simulink model "filter_music"  (R2021a)
settings: Solver=FixedStepDiscrete  StartTime=0.0  StopTime=inf  RelTol=1e-3
undefined symbols (not defined in the file or in its folder): fdesignblkfcn, gcbh
libraries: dspfdesign x2, dspsnks4 x1, dspvision x1
(part 2 of 2)

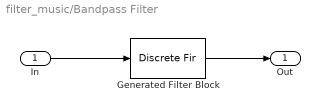
== system filter_music/Bandpass Filter ==
  In : Inport
  Generated Filter Block : DiscreteFir  Tag=BlockMethodSubSystem  Coefficients=[-0.000605180765563559896 -0.000235381781177703146 -0.000262859375971625413 -0.000278554889448817417 -0.000279923053767988173 -0.000265464035195501331 -0.000234716056378071693 -0.00018863467570875262 -0.000129411281477895067 -6.06366503102824512e-05 1.31467495266928401e-05 8.65511069714545132e-05 0.000154034385313488062 0.000210145628121449752 0.000250253378986492556 0.00027071164836725976 0.000269490837798465311 0.000246231290949470159 0.000202784352817899423 0.000143028939846710291 7.29851468422456316e-05 -4.77348731589156425e-08 -6.79070740966332198e-05 -0.000122541384684050962 -0.000155931925683581134 -0.000160955543706951999 -0.000132226172829594377 -6.83521227724636759e-05 2.96378115559616279e-05 0.000160133019832697597 0.000313569795262432708 0.000481870213809313969 0.000652141561601816229 0.000811036194270708792 0.000944251143223556614 0.00103811317126550613 0.00108045816269594945 0.00106184513278247605 0.000976405444503380244 0.00082256507615554122 0.000603383089157199072 0.000326581850271807439 4.30229332145489322e-06 -0.000347509148140041164 -0.000709960328759635549 -0.00106252114048841937 -0.00138437477114929076 -0.00165591825323341529 -0.00185992926996901738 -0.00198287607906476315 -0.00201592256171890302 -0.00195586315981783384 -0.00180507449704414048 -0.00157138964197742789 -0.00126771264216854322 -0.000911677520776701445 -0.000523426256061187674 -0.000124603742469066113 0.000262166881930523115 0.00061678380216169859 0.000920925730041676697 0.0011607996965117013 0.00132708911283209246 0.00141590960857993289 0.00142864204842689199 0.00137169545143854825 0.00125574284285703266 0.00109477510338883361 0.000904879511926304876 0.00070287872131849006 0.000504967982929463671 0.000325453791699786691 0.000175792867800047452 6.37979729521747317e-05 -6.78212542151071728e-06 -3.64090327009696142e-05 -2.93132352749527577e-05 7.10364132435301075e-06 6.31354581538463882e-05 0.000127627008729503587 0.000189328520858482891 0.000237969883486319108 0.000265138541684875443 0.000264854787163768164 0.000234581092845862979 0.00017485918044263192 8.92504407498085451e-05 -1.55906822884784904e-05 -0.000131442770007978067 -0.00024855850135476051 -0.000357255458734658665 -0.000448464748990436764 -0.000514815634287659135 -0.000551228314512786977 -0.000555453484683462984 -0.000528225669558642693 -0.000473150348547238578 -0.000396334954072101626 -0.000305796015337770548 -0.000210708853438425523 -0.00012045061728521669 -4.37072089313232244e-05 1.23630628756550677e-05 4.27142101961259989e-05 4.49781553983374631e-05 1.9660819291976721e-05 -2.99127335878764909e-05 -9.80525281223114018e-05 -0.000177090847882267245 -0.00025819999365800085 -0.000332283691101674156 -0.000390876997623911665 -0.000426702885764895128 -0.000434764417987566461 -0.000412523468574856414 -0.000360143401753243897 -0.000280728629105348273 -0.0001796370023316761 -6.43780874097095831e-05 5.64046858719952703e-05 0.000173558948389901152 0.000278390928633116851 0.000363384696453391285 0.000422902032819955044 0.000453692365489637096 0.000455170057780033112 0.000429423377421828936 0.000380926372577061018 0.000316118651487450845 0.000242744677068970638 0.000169102399701490135 0.00010315597790109865 5.18457342326022103e-05 2.03957843541542314e-05 1.1834016995465772e-05 2.66453462442806933e-05 6.28868593623271019e-05 0.000116297826640652144 0.000180744685678951243 0.000248860486110872041 0.000312892640430147931 0.000365219026156458199 0.000399385636178222012 0.000410560159007349143 0.000396034523223016749 0.000355634528508955259 0.000291517013176819859 0.000208166915657288272 0.000111812151609713912 9.94064949812921566e-06 -8.94947208903917678e-05 -0.000178824590337025744 -0.000251393008747853987 -0.000302179769701022992 -0.000328265064184263917 -0.000329135996664805901 -0.000306672623430111159 -0.000264957328971117238 -0.000209833026406665735 -0.000148369133699592984 -8.80772297146796822e-05 -3.6207021158947418e-05 9.85174473132223272e-07 1.88151056810751905e-05 1.47474060914241016e-05 ...(+44349 chars)]  InputProcessing=Columns as channels (frame based)
  Out : Outport  VectorParamsAs1DForOutWhenUnconnected=off
  wires:
  In/1 -> Generated Filter Block/1
  Generated Filter Block/1 -> Out/1
